simulink model "Parallelschwingkreis"  (R2021b)
settings: Solver=ode1  StartTime=0.0  StopTime=10.0  FixedStep=0.00001  RelTol=1e-3
settings Model: Creator=the_main_notebook  LastModifiedBy=the_main_notebook

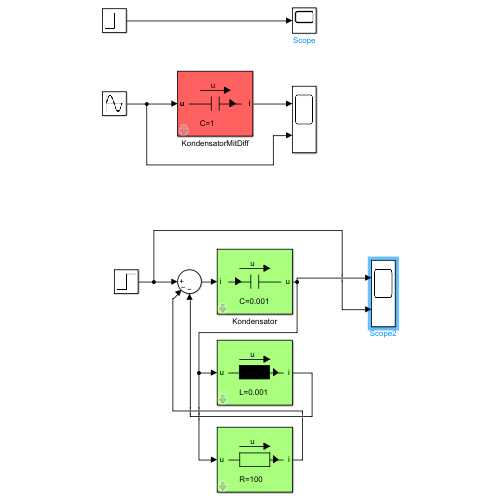
[thumbnail: Simulink's stored preview of the top-level diagram]
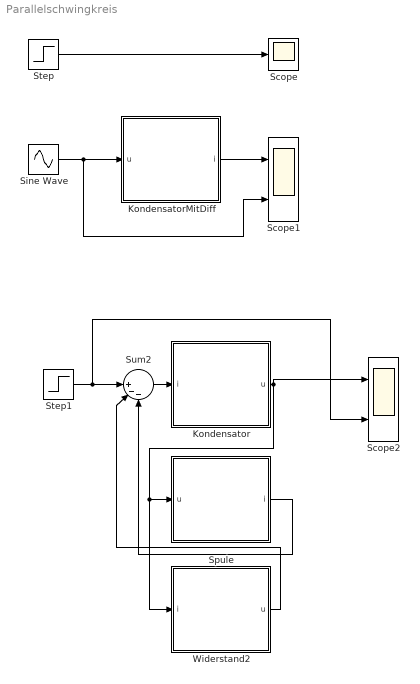
== system Parallelschwingkreis ==
  Kondensator : Subsystem  mask{C=1E-3}
      mask prompts: C "Kappazität C [F]"
      mask help:
      | Kapazität
      | Eingang ist u, Ausgang ist i.
      | i=1/C * integral(u)
      mask Display:
      | plot(0,0)
      | plot(100,100)
      | plot([0 0],[1 1]) %Umschalten auf dicke Linien
      | %patch([30 30 70 70 30],[40 60 60 40 40],[0,0,0])
      | plot([45 45],[40 60])
      | plot([55 55],[40 60])
      | plot([15 45],[50 50])
      | patch([25,32,25],[45,50,55],[0,0,0])
      | plot([55 85],[50 50])
      | plot([30 70],[70 70])
      | patch([63 70 63],[65 70 75], [0,0,0])
      | text(45,80,['u'])
      | 
      | text(30,20,['C=',num2str(C)])
      | 
      | 
      | 
      | port_label ('output',1,'u')
      | port_label ('input',1,'i')
  KondensatorMitDiff : Subsystem  mask{C=1}
      mask prompts: C "Kappazität C [F]"
      mask help:
      | Kapazität
      | Eingang ist u, Ausgang ist i.
      | i=C*u'
      | Wegen Diff-Block nicht für jeden Solver geeignet.
      mask Display:
      | plot(0,0)
      | plot(100,100)
      | plot([0 0],[1 1]) %Umschalten auf dicke Linien
      | %patch([30 30 70 70 30],[40 60 60 40 40],[0,0,0])
      | plot([45 45],[40 60])
      | plot([55 55],[40 60])
      | plot([15 45],[50 50])
      | patch([70,77,70],[45,50,55],[0,0,0])
      | plot([55 85],[50 50])
      | plot([30 70],[70 70])
      | patch([63 70 63],[65 70 75], [0,0,0])
      | text(45,80,['u'])
      | 
      | text(30,20,['C=',num2str(C)])
      | 
      | 
      | 
      | port_label ('output',1,'i')
      | port_label ('input',1,'u')
  Scope : Scope
  Scope1 : Scope  NumInputPorts=2
  Scope2 : Scope  NumInputPorts=2
  Sine Wave : Sin  SampleTime=0
  Spule : Subsystem  mask{L=1E-3}
      mask prompts: L "Induktivität L [H]"
      mask help:
      | Induktivität:
      | Eingang ist u, Ausgang ist i.
      mask Display:
      | plot(0,0)
      | plot(100,100)
      | plot([0 0],[1 1]) %Umschalten auf dicke Linien
      | patch([30 30 70 70 30],[40 60 60 40 40],[0,0,0])
      | plot([15 30],[50 50])
      | patch([75,82,75],[45,50,55],[0,0,0])
      | plot([70 88],[50 50])
      | plot([30 70],[70 70])
      | patch([63 70 63],[65 70 75], [0,0,0])
      | text(45,80,['u'])
      | 
      | text(30,20,['L=',num2str(L)])
      | 
      | 
      | 
      | port_label ('output',1,'i')
      | port_label ('input',1,'u')
  Step : Step  SampleTime=0
  Step1 : Step  SampleTime=0
  Sum2 : Sum  Inputs=||+--
  Widerstand2 : Subsystem  mask{R=100}
      mask prompts: R "Widerstand [Ohm]"
      mask help: Ohm'scher Widerstand, Eingang ist u, Ausgang ist i.
      mask Display:
      | plot(0,0)
      | plot(100,100)
      | plot([0 0],[1 1]) %Umschalten auf dicke Linien
      | plot([30 30 70 70 30],[40 60 60 40 40])
      | plot([15 30],[50 50])
      | patch([75,82,75],[45,50,55],[0,0,0])
      | plot([70 88],[50 50])
      | plot([30 70],[70 70])
      | patch([63 70 63],[65 70 75], [0,0,0])
      | text(45,80,['u'])
      | 
      | text(30,20,['R=',num2str(R)])
      | 
      | 
      | 
      | port_label ('output',1,'i')
      | port_label ('input',1,'u')
  wires:
  Step/1 -> Scope/1
  KondensatorMitDiff/1(i) -> Scope1/1
  Sine Wave/1 -> Scope1/2, KondensatorMitDiff/1(u)
  Sum2/1 -> Kondensator/1(i)
  Kondensator/1(u) -> Widerstand2/1(i), Spule/1(u), Scope2/1
  Spule/1(i) -> Sum2/3
  Widerstand2/1(u) -> Sum2/2
  Step1/1 -> Scope2/2, Sum2/1

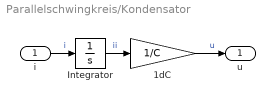
== system Parallelschwingkreis/Kondensator ==
  i : Inport
  1dC : Gain  Gain=1/C
  Integrator : Integrator
  u : Outport  VectorParamsAs1DForOutWhenUnconnected=off
  wires:
  Integrator/1 -> 1dC/1  "ii"
  1dC/1 -> u/1  "u"
  i/1 -> Integrator/1  "i"

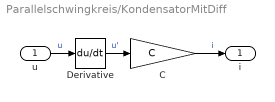
== system Parallelschwingkreis/KondensatorMitDiff ==
  u : Inport
  C : Gain  Gain=C
  Derivative : Derivative
  i : Outport  VectorParamsAs1DForOutWhenUnconnected=off
  wires:
  Derivative/1 -> C/1  "u'"
  C/1 -> i/1  "i"
  u/1 -> Derivative/1  "u"

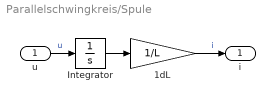
== system Parallelschwingkreis/Spule ==
  u : Inport
  1dL : Gain  Gain=1/L
  Integrator : Integrator
  i : Outport  VectorParamsAs1DForOutWhenUnconnected=off
  wires:
  Integrator/1 -> 1dL/1
  1dL/1 -> i/1  "i"
  u/1 -> Integrator/1  "u"

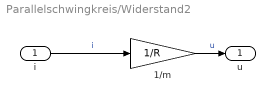
== system Parallelschwingkreis/Widerstand2 ==
  i : Inport
  1/m : Gain  Gain=1/R
  u : Outport  VectorParamsAs1DForOutWhenUnconnected=off
  wires:
  1/m/1 -> u/1  "u"
  i/1 -> 1/m/1  "i"
